simulink model "moteur_hacheur"  (R2024a)
settings: Solver=VariableStepAuto  StartTime=0.0  StopTime=0.2  RelTol=1e-3
values from neighbouring files (symbols this model uses):
  Co = 2.4e-2    (= 0.024)    [moteur_avec_hacheur.m]
  f = (5.3e-3/1e3)*30/pi    (= 5.06112719032e-05)    [moteur_avec_hacheur.m]
  J = 8.3e-5    (= 8.3e-05)    [moteur_avec_hacheur.m]
  Kphi = 0.127    [moteur_avec_hacheur.m]
  L = 2.2e-3    (= 0.0022)    [moteur_avec_hacheur.m]
  R = 1.52    [moteur_avec_hacheur.m]
  Rch = 10    [moteur_avec_hacheur.m]
  U = 48    [moteur_avec_hacheur.m]
settings Model: Creator=mguerchon01  LastModifiedBy=magic

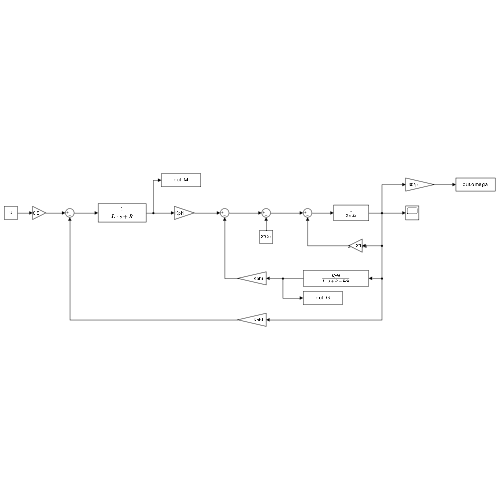
[thumbnail: Simulink's stored preview of the top-level diagram]
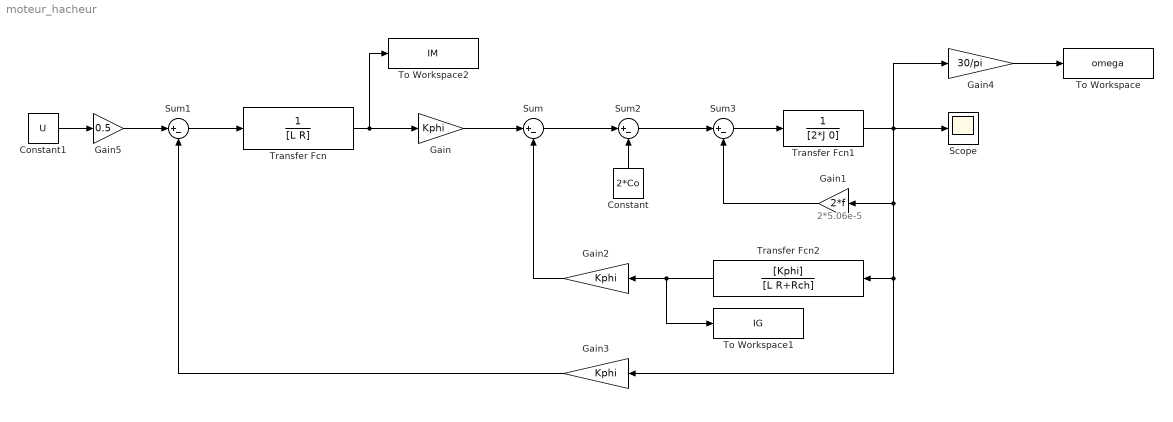
== system moteur_hacheur ==
  note: 2*5.06e-5
  Constant : Constant  Value=2*Co
  Constant1 : Constant  Value=U
  Gain : Gain  Gain=Kphi
  Gain1 : Gain  Gain=2*f
  Gain2 : Gain  Gain=Kphi
  Gain3 : Gain  Gain=Kphi
  Gain4 : Gain  Gain=30/pi
  Gain5 : Gain  Gain=0.5
  Scope : Scope
  Sum{,1..3} (4 alike) : Sum  Inputs=|+-
  To Workspace : ToWorkspace  VariableName=omega  SaveFormat=Timeseries  SampleTime=-1
  To Workspace1 : ToWorkspace  VariableName=IG  SaveFormat=Timeseries  SampleTime=-1
  To Workspace2 : ToWorkspace  VariableName=IM  SaveFormat=Timeseries  SampleTime=-1
  Transfer Fcn : TransferFcn  Denominator=[L R]
  Transfer Fcn1 : TransferFcn  Denominator=[2*J 0]
  Transfer Fcn2 : TransferFcn  Numerator=[Kphi]  Denominator=[L R+Rch]
  wires:
  Transfer Fcn/1 -> To Workspace2/1, Gain/1
  Sum1/1 -> Transfer Fcn/1
  Gain/1 -> Sum/1
  Constant/1 -> Sum2/2
  Sum2/1 -> Sum3/1
  Sum/1 -> Sum2/1
  Sum3/1 -> Transfer Fcn1/1
  Transfer Fcn1/1 -> Gain4/1, Scope/1, Gain3/1, Transfer Fcn2/1, Gain1/1
  Gain1/1 -> Sum3/2
  Transfer Fcn2/1 -> To Workspace1/1, Gain2/1
  Gain2/1 -> Sum/2
  Gain3/1 -> Sum1/2
  Gain4/1 -> To Workspace/1
  Gain5/1 -> Sum1/1
  Constant1/1 -> Gain5/1
